simulink model "YCrCb_Color_Component_AutoThresholding"  (R2016a)
settings: Solver=VariableStepAuto  StartTime=0.0  StopTime=10.0  RelTol=1e-3
undefined symbols (not defined in the file): Rec, SDTV
libraries: visionstatistics x6, visionconversions x4, visionsinks x3, visionsources x1
settings Model: Creator=YASARA  LastModifiedBy=YASARA

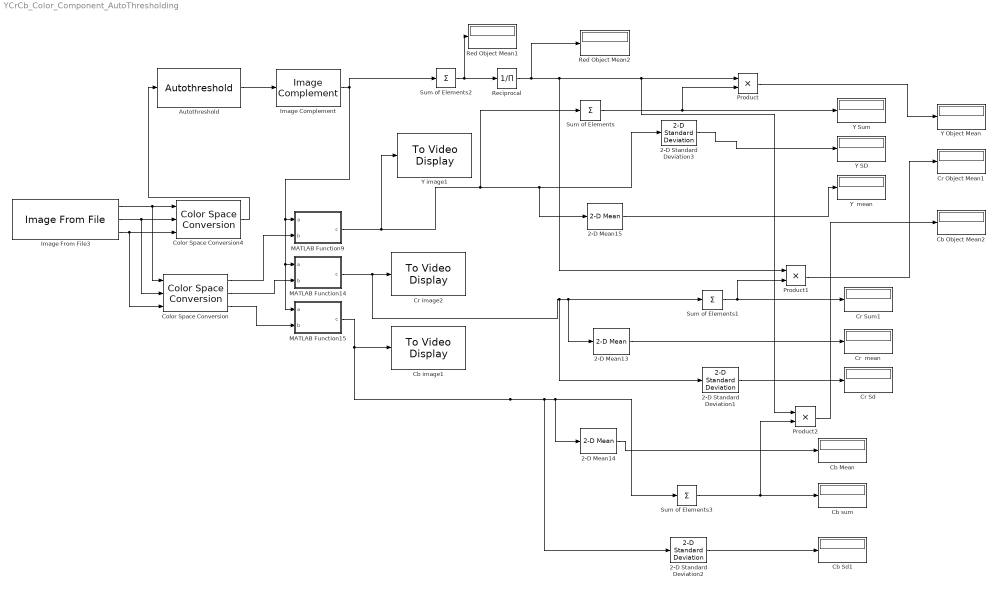
== system YCrCb_Color_Component_AutoThresholding ==
  2-D Mean13 : visionstatistics/2-D Mean  run=off  reset_popup=None  directionMode=Entire input  dimension=1  treatSBRowAsCol=on  roiEnable=off  roiType=Rectangles  roiPortion=Entire ROI  roiOutput=Individual statistics for each ROI  roiFlag=off  outputDataTypeStr=Inherit: Same as accumulator  outputLastDataTypeStr=Inherit: Same as accumulator  outputMin=[]  outputMax=[]  accumMode=Binary point scaling  accumWordLength=32  accumFracLength=0  accumDataTypeStr=fixdt([],32,0)  accumLastDataTypeStr=fixdt([],32,0)  roundingMode=Floor  overflowMode=off
  2-D Mean14 : visionstatistics/2-D Mean  run=off  reset_popup=None  directionMode=Entire input  dimension=1  treatSBRowAsCol=on  roiEnable=off  roiType=Rectangles  roiPortion=Entire ROI  roiOutput=Individual statistics for each ROI  roiFlag=off  outputDataTypeStr=Inherit: Same as accumulator  outputLastDataTypeStr=Inherit: Same as accumulator  outputMin=[]  outputMax=[]  accumMode=Binary point scaling  accumWordLength=32  accumFracLength=0  accumDataTypeStr=fixdt([],32,0)  accumLastDataTypeStr=fixdt([],32,0)  roundingMode=Floor  overflowMode=off
  2-D Mean15 : visionstatistics/2-D Mean  run=off  reset_popup=None  directionMode=Entire input  dimension=1  treatSBRowAsCol=on  roiEnable=off  roiType=Rectangles  roiPortion=Entire ROI  roiOutput=Individual statistics for each ROI  roiFlag=off  outputDataTypeStr=Inherit: Same as accumulator  outputLastDataTypeStr=Inherit: Same as accumulator  outputMin=[]  outputMax=[]  accumMode=Binary point scaling  accumWordLength=32  accumFracLength=0  accumDataTypeStr=fixdt([],32,0)  accumLastDataTypeStr=fixdt([],32,0)  roundingMode=Floor  overflowMode=off
  2-D Standard Deviation1 : visionstatistics/2-D Standard Deviation  run=off  reset_popup=None  directionMode=Entire input  dimension=1  treatSBRowAsCol=on  roiEnable=off  roiType=Rectangles  roiPortion=Entire ROI  roiOutput=Individual statistics for each ROI  roiFlag=off
  2-D Standard Deviation2 : visionstatistics/2-D Standard Deviation  run=off  reset_popup=None  directionMode=Entire input  dimension=1  treatSBRowAsCol=on  roiEnable=off  roiType=Rectangles  roiPortion=Entire ROI  roiOutput=Individual statistics for each ROI  roiFlag=off
  2-D Standard Deviation3 : visionstatistics/2-D Standard Deviation  run=off  reset_popup=None  directionMode=Entire input  dimension=1  treatSBRowAsCol=on  roiEnable=off  roiType=Rectangles  roiPortion=Entire ROI  roiOutput=Individual statistics for each ROI  roiFlag=off
  Autothreshold : visionconversions/Autothreshold  operator=>  threshOut=off  effMetricOut=off  userDefinedRange=off  umin=0  umax=255  outOfRngOpt=Warn and saturate  scaleThreshold=off  scaleFactor=1  P1Mode=Specify word length  P1WordLength=32  P1FracLength=30  P2Mode=Specify word length  P2WordLength=32  P2FracLength=22  P3Mode=Specify word length  P3WordLength=32  P3FracLength=14  P4Mode=Binary point scaling  P4WordLength=32  P4FracLength=15  Q1Mode=Specify word length  Q1WordLength=32  Q1FracLength=16  EMMode=Specify word length  EMWordLength=16  EMFracLength=14  roundingMode=Floor  overflowMode=off
  Cb Mean : Display
  Cb Object Mean2 : Display
  Cb Sd1 : Display
  Cb image1 : visionsinks/To Video Display  windowSizeMode=Normal  openAtMdlStart=on  fullScreen=off  videoWindowX=252  videoWindowY=213  saveWindowSize=off  videoWindowWidth=512  videoWindowHeight=384  inputColorFormat=RGB  inputType=Obsolete  imagePorts=One multidimensional signal  OutputDevice=On-screen video monitor  dataOrg=Column-major  isWindowOpen=off
  Cb sum : Display
  Color Space Conversion : visionconversions/Color Space  Conversion  conversion=Obsolete  conversionActive=R'G'B' to Y'CbCr  wp_str=D65  rec=Rec. 601 (SDTV)  sys=1125/60/2:1  imagePorts=Separate color signals
  Color Space Conversion4 : visionconversions/Color Space  Conversion  conversion=Obsolete  conversionActive=R'G'B' to intensity  wp_str=D65  rec=Rec. 601 (SDTV)  sys=1125/60/2:1  imagePorts=Separate color signals
  Cr  mean : Display
  Cr Object Mean1 : Display
  Cr Sd : Display
  Cr Sum1 : Display
  Cr image2 : visionsinks/To Video Display  windowSizeMode=Normal  openAtMdlStart=on  fullScreen=off  videoWindowX=252  videoWindowY=213  saveWindowSize=off  videoWindowWidth=512  videoWindowHeight=384  inputColorFormat=RGB  inputType=Obsolete  imagePorts=One multidimensional signal  OutputDevice=On-screen video monitor  dataOrg=Column-major  isWindowOpen=off
  Image Complement : visionconversions/Image Complement
  Image From File3 : visionsources/Image From File  Tag=vipblks_nd  FileName=C:\Users\YASARA\Desktop\FRY_Docu\tea\teaxb.jpg  imagePorts=Separate color signals  Ts=1  ImageDataType=double  Signed=on  WordLength=16  sdImageDataType=uint(8)  FractionLengthMode=User-defined  FractionLength=15  OutPortLabels=R|G|B
  MATLAB Function14 : MATLAB Function  TreatAsAtomicUnit=on
  MATLAB Function15 : MATLAB Function  TreatAsAtomicUnit=on
  MATLAB Function9 : MATLAB Function  TreatAsAtomicUnit=on
  Product : Product
  Product1 : Product
  Product2 : Product
  Reciprocal : Product  Inputs=/  OutDataTypeStr=double  SaturateOnIntegerOverflow=on  RndMeth=Zero
  Red Object Mean1 : Display
  Red Object Mean2 : Display
  Sum of Elements{,1..3} (4 alike) : Sum  Inputs=+
  Y  mean : Display
  Y Object Mean : Display
  Y SD : Display
  Y Sum : Display
  Y image1 : visionsinks/To Video Display  windowSizeMode=Normal  openAtMdlStart=on  fullScreen=off  videoWindowX=252  videoWindowY=213  saveWindowSize=off  videoWindowWidth=512  videoWindowHeight=384  inputColorFormat=RGB  inputType=Obsolete  imagePorts=One multidimensional signal  OutputDevice=On-screen video monitor  dataOrg=Column-major  isWindowOpen=off
  wires:
  Image From File3/1 -> Color Space Conversion/1, Color Space Conversion4/1
  Image From File3/2 -> Color Space Conversion/2, Color Space Conversion4/2
  Image From File3/3 -> Color Space Conversion/3, Color Space Conversion4/3
  Autothreshold/1 -> Image Complement/1
  2-D Mean15/1 -> Y  mean/1
  2-D Mean13/1 -> Cr  mean/1
  Sum of Elements/1 -> Product/2, Y Sum/1
  MATLAB Function9/1(c) -> Y image1/1, 2-D Mean15/1, 2-D Standard Deviation3/1, Sum of Elements/1
  2-D Standard Deviation3/1 -> Y SD/1
  2-D Standard Deviation1/1 -> Cr Sd/1
  MATLAB Function14/1(c) -> 2-D Standard Deviation1/1, 2-D Mean13/1, Sum of Elements1/1, Cr image2/1
  Sum of Elements3/1 -> Product2/2, Cb sum/1
  2-D Standard Deviation2/1 -> Cb Sd1/1
  MATLAB Function15/1(c) -> Cb image1/1, 2-D Standard Deviation2/1, 2-D Mean14/1, Sum of Elements3/1
  Sum of Elements2/1 -> Red Object Mean1/1, Reciprocal/1
  Product/1 -> Y Object Mean/1
  Sum of Elements1/1 -> Product1/2, Cr Sum1/1
  Product1/1 -> Cr Object Mean1/1
  2-D Mean14/1 -> Cb Mean/1
  Product2/1 -> Cb Object Mean2/1
  Reciprocal/1 -> Red Object Mean2/1, Product2/1, Product/1, Product1/1
  Image Complement/1 -> MATLAB Function15/1(a), MATLAB Function14/1(a), MATLAB Function9/1(a), Sum of Elements2/1
  Color Space Conversion/1 -> MATLAB Function9/2(b)
  Color Space Conversion/2 -> MATLAB Function14/2(b)
  Color Space Conversion/3 -> MATLAB Function15/2(b)
  Color Space Conversion4/1 -> Autothreshold/1

== matlab function YCrCb_Color_Component_AutoThresholding/MATLAB Function14 ==
  data: a input; b input; c output
function c = fcn(a,b)
%#codegen
c=a.*b;
return

== matlab function YCrCb_Color_Component_AutoThresholding/MATLAB Function15 ==
  data: a input; b input; c output
function c = fcn(a,b)
%#codegen
c=a.*b;
return

== matlab function YCrCb_Color_Component_AutoThresholding/MATLAB Function9 ==
  data: a input; b input; c output
function c = fcn(a,b)
%#codegen
c=a.*b;
return
